simulink model "lab11question2"  (Simulink 6.6)
settings: Solver=ode45  StartTime=0.0  StopTime=100.0  RelTol=1e-3
InitFcn:
  | K = 1
  | 
  | gs_den = conv([1 1],conv([1 3],[1 6 13]));
settings Model: Creator=Adriano  LastModifiedBy=Adriano

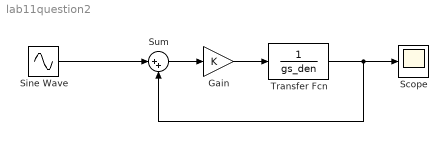
== system lab11question2 ==
  Gain : Gain  Gain=K
  Scope : Scope
  Sine Wave : Sin  Frequency=3  SampleTime=0
  Sum : Sum  Inputs=|++
  Transfer Fcn : TransferFcn  Denominator=gs_den
  wires:
  Sine Wave/1 -> Sum/1
  Sum/1 -> Gain/1
  Gain/1 -> Transfer Fcn/1
  Transfer Fcn/1 -> Sum/2, Scope/1
